simulink model "audio_dan"  (R2014a)
settings: Solver=FixedStepDiscrete  StartTime=0.0  StopTime=inf  FixedStep=0.00025  RelTol=1e-3
libraries: xpcethercatlib x12, slrtlib x4, simulink x1
settings Model: xpc_rtwmakecfg_data=_xpcethercatlib_  SimulationMode=external  BufferReuse=off  Creator=drl  LastModifiedBy=drl
settings SolverCC: EnableConcurrentExecution=on  ConcurrentTasks=on
settings OptimizationCC: BlockReduction=off  OptimizeBlockIOStorage=off  BufferReuse=off  GlobalBufferReuse=off  ExpressionFolding=off  LocalBlockOutputs=off
settings HardwareCC: ProdIntDivRoundTo=Zero  ProdEndianess=LittleEndian  ProdHWDeviceType=Generic->32-bit x86 compatible
settings RTWCC: SystemTargetFile=slrt.tlc  TemplateMakefile=slrt_default_tmf  Description=Simulink Real-Time  ProcessScript=slrt_make_rtw_hook  RTWCompilerOptimization=On
settings SimulinkRealTimeCC: GeneratePreprocessorConditionals=Disable all  EnableShiftOperators=on

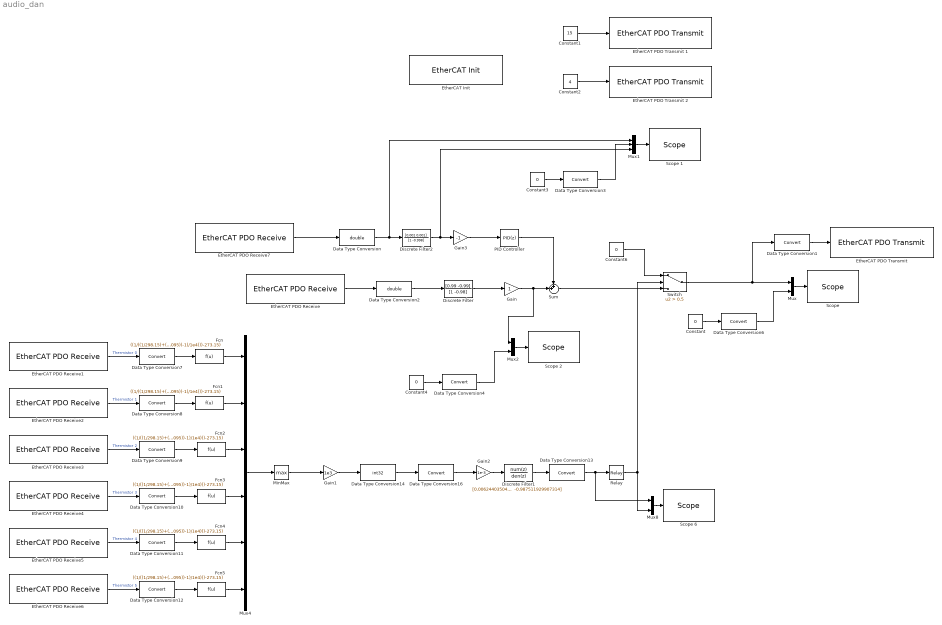
== system audio_dan ==
  Constant : Constant  Value=0  OutDataTypeStr=Inherit: Inherit via back propagation
  Constant1 : Constant  Value=15  OutDataTypeStr=Inherit: Inherit via back propagation  SampleTime=-1
  Constant2 : Constant  Value=4  OutDataTypeStr=Inherit: Inherit via back propagation  SampleTime=-1
  Constant3 : Constant  Value=0  OutDataTypeStr=Inherit: Inherit via back propagation
  Constant4 : Constant  Value=0  OutDataTypeStr=Inherit: Inherit via back propagation
  Constant6 : Constant  Value=0
  Data Type Conversion : DataTypeConversion  OutDataTypeStr=double
  Data Type Conversion{1,3..4,6..13,16} (12 alike) : DataTypeConversion
  Data Type Conversion14 : DataTypeConversion  OutDataTypeStr=int32
  Data Type Conversion2 : DataTypeConversion  OutDataTypeStr=double
  Discrete Filter : DiscreteFilter  Numerator=[0.99 -0.99]  Denominator=[1 -0.98]  a0EqualsOne=on
  Discrete Filter1 : DiscreteFilter  Numerator="[0.006244035046343   0.006244035046343]"  Denominator="[1.000000000000000  -0.987511929907314]"  a0EqualsOne=on
  Discrete Filter2 : DiscreteFilter  Numerator=[0.001 0.001]  Denominator=[1 -0.998]  a0EqualsOne=on
  "EtherCAT Init " : xpcethercatlib/EtherCAT Init   Priority=0  config_file=C:\Users\drl\Documents\MATLAB\eni_elmo_medulla_4khz.xml  device_id=0  pci_bus=4  pci_slot=0  enaDebug=on  enaDC=on  errLink=off  masterDbg=off  stateChgDbg=off  baseClock=off  masterCfg=off  logFile='c:\dbglog.txt'  sample_time=0.000250
  EtherCAT PDO Receive : xpcethercatlib/EtherCAT PDO Receive  Priority=2  sig_name=Drive 1 (Elmo Drive).Inputs.Analog Input 1  sig_offset=1144  sig_type=int16  type_size=16  sig_dim=1  device_id=0  sample_time=0.000250
  EtherCAT PDO Receive1 : xpcethercatlib/EtherCAT PDO Receive  Priority=2  sig_name=Box 2 (ATRIAS 2.1 Leg (Medulla 1.5)).Thermistors.Thermistor 0  sig_offset=808  sig_type=uint16  type_size=16  sig_dim=1  device_id=0  sample_time=0.000250
  EtherCAT PDO Receive2 : xpcethercatlib/EtherCAT PDO Receive  Priority=2  sig_name=Box 2 (ATRIAS 2.1 Leg (Medulla 1.5)).Thermistors.Thermistor 1  sig_offset=824  sig_type=uint16  type_size=16  sig_dim=1  device_id=0  sample_time=0.000250
  EtherCAT PDO Receive3 : xpcethercatlib/EtherCAT PDO Receive  Priority=2  sig_name=Box 2 (ATRIAS 2.1 Leg (Medulla 1.5)).Thermistors.Thermistor 2  sig_offset=840  sig_type=uint16  type_size=16  sig_dim=1  device_id=0  sample_time=0.000250
  EtherCAT PDO Receive4 : xpcethercatlib/EtherCAT PDO Receive  Priority=2  sig_name=Box 2 (ATRIAS 2.1 Leg (Medulla 1.5)).Thermistors.Thermistor 3  sig_offset=856  sig_type=uint16  type_size=16  sig_dim=1  device_id=0  sample_time=0.000250
  EtherCAT PDO Receive5 : xpcethercatlib/EtherCAT PDO Receive  Priority=2  sig_name=Box 2 (ATRIAS 2.1 Leg (Medulla 1.5)).Thermistors.Thermistor 4  sig_offset=872  sig_type=uint16  type_size=16  sig_dim=1  device_id=0  sample_time=0.000250
  EtherCAT PDO Receive6 : xpcethercatlib/EtherCAT PDO Receive  Priority=2  sig_name=Box 2 (ATRIAS 2.1 Leg (Medulla 1.5)).Thermistors.Thermistor 5  sig_offset=888  sig_type=uint16  type_size=16  sig_dim=1  device_id=0  sample_time=0.000250
  EtherCAT PDO Receive7 : xpcethercatlib/EtherCAT PDO Receive  Priority=2  sig_name=Drive 1 (Elmo Drive).Inputs.Position actual value  sig_offset=1064  sig_type=int32  type_size=32  sig_dim=1  device_id=0  sample_time=0.000250
  "EtherCAT PDO Transmit " : xpcethercatlib/EtherCAT PDO Transmit   Priority=3  sig_name=Drive 1 (Elmo Drive).Outputs.Target Torque  sig_offset=1064  sig_type=int16  type_size=16  sig_dim=1  device_id=0  sample_time=0.000250
  EtherCAT PDO Transmit 1 : xpcethercatlib/EtherCAT PDO Transmit   Priority=3  sig_name=Drive 1 (Elmo Drive).Outputs.Control word  sig_offset=1080  sig_type=uint16  type_size=16  sig_dim=1  device_id=0  sample_time=0.000250
  EtherCAT PDO Transmit 2 : xpcethercatlib/EtherCAT PDO Transmit   Priority=3  sig_name=Drive 1 (Elmo Drive).Outputs.Mode of operation  sig_offset=1096  sig_type=int8  type_size=8  sig_dim=1  device_id=0  sample_time=0.000250
  Fcn{,1..5} (6 alike) : Fcn  Expr=((1/((1/298.15)+(1/3988)*log(4700/((3.26/((u-172)*2.7/4095))-1)/1e4)))-273.15)
  Gain : Gain
  Gain1 : Gain  Gain=1e3
  Gain2 : Gain  Gain=1e-3
  Gain3 : Gain  Gain=-1
  MinMax : MinMax  Function=max
  Mux : Mux  Inputs=2
  Mux1 : Mux  Inputs=3
  Mux2 : Mux  Inputs=2
  Mux4 : Mux  Inputs=6
  Mux8 : Mux  Inputs=2
  PID Controller : simulink/Continuous/PID Controller  Controller=PID  TimeDomain=Discrete-time  SampleTime=-1  IntegratorMethod=Forward Euler  FilterMethod=Forward Euler  Form=Parallel  P=0.01  I=0  D=0.01  N=100  InitialConditionSource=internal  InitialConditionForIntegrator=0  InitialConditionForFilter=0  ExternalReset=none  LimitOutput=on  UpperSaturationLimit=200  LowerSaturationLimit=-200  LinearizeAsGain=on  AntiWindupMode=none  Kb=1  TrackingMode=off  Kt=1  PParamMin=[]  PParamMax=[]  IParamMin=[]  IParamMax=[]  DParamMin=[]  DParamMax=[]  NParamMin=[]  NParamMax=[]  KbParamMin=[]  KbParamMax=[]  KtParamMin=[]  KtParamMax=[]  POutMin=[]  POutMax=[]  IOutMin=[]  IOutMax=[]  DOutMin=[]  DOutMax=[]  NOutMin=[]  NOutMax=[]  KbOutMin=[]  KbOutMax=[]  KtOutMin=[]  KtOutMax=[]  IntegratorOutMin=[]  IntegratorOutMax=[]  FilterOutMin=[]  FilterOutMax=[]  SumOutMin=[]  SumOutMax=[]  SumI1OutMin=[]  SumI1OutMax=[]  SumI2OutMin=[]  SumI2OutMax=[]  SumI3OutMin=[]  SumI3OutMax=[]  SumDOutMin=[]  SumDOutMax=[]  SaturationOutMin=[]  SaturationOutMax=[]  IntegratorContinuousStateAttributes=''  IntegratorStateMustResolveToSignalObject=off  IntegratorRTWStateStorageClass=Auto  FilterContinuousStateAttributes=''  FilterStateMustResolveToSignalObject=off  FilterRTWStateStorageClass=Auto
  Relay : Relay  OnSwitchValue=80  OffSwitchValue=60
  "Scope " : slrtlib/Displays and Logging/Scope   scopeno=1  scopetype=Target  autostart=on  viewmode=Graphical rolling  formatstr='%15.6f'  grid=on  ylimits=[0,0]  nosamples=1000  noprepostsamples=0  interleave=1  triggermode=FreeRun  triggersignal=1  trigsignalfromport=off  triggerlevel=0.0  triggerslope=Either  triggerscope=1  triggersample=0  filename=data.dat  mode=Lazy  writesize=512  autorestart=off  dynamicfilemode=off  maxwritefilesize=512*1024^2
  Scope 1 : slrtlib/Displays and Logging/Scope   scopeno=3  scopetype=Target  autostart=on  viewmode=Graphical rolling  formatstr='%15.6f'  grid=on  ylimits=[0,0]  nosamples=1000  noprepostsamples=0  interleave=1  triggermode=FreeRun  triggersignal=1  trigsignalfromport=off  triggerlevel=0.0  triggerslope=Either  triggerscope=1  triggersample=0  filename=data.dat  mode=Lazy  writesize=512  autorestart=off  dynamicfilemode=off  maxwritefilesize=512*1024^2
  Scope 2 : slrtlib/Displays and Logging/Scope   scopeno=4  scopetype=Target  autostart=on  viewmode=Graphical rolling  formatstr='%15.6f'  grid=on  ylimits=[0,0]  nosamples=1000  noprepostsamples=0  interleave=1  triggermode=FreeRun  triggersignal=1  trigsignalfromport=off  triggerlevel=0.0  triggerslope=Either  triggerscope=1  triggersample=0  filename=data.dat  mode=Lazy  writesize=512  autorestart=off  dynamicfilemode=off  maxwritefilesize=512*1024^2
  Scope 6 : slrtlib/Displays and Logging/Scope   scopeno=2  scopetype=Target  autostart=on  viewmode=Numerical  formatstr='%f'  grid=on  ylimits=[0,0]  nosamples=100  noprepostsamples=0  interleave=1  triggermode=FreeRun  triggersignal=1  trigsignalfromport=off  triggerlevel=0.0  triggerslope=Either  triggerscope=2  triggersample=0  filename=data.dat  mode=Lazy  writesize=512  autorestart=off  dynamicfilemode=off  maxwritefilesize=512*1024^2
  Sum : Sum  Inputs=++|
  Switch : Switch  Criteria=u2 > Threshold  Threshold=0.5
  wires:
  Mux/1 -> "Scope "/1
  Data Type Conversion1/1 -> "EtherCAT PDO Transmit "/1
  Constant1/1 -> EtherCAT PDO Transmit 1/1
  Constant2/1 -> EtherCAT PDO Transmit 2/1
  EtherCAT PDO Receive6/1 -> Data Type Conversion12/1  "Thermistor 5"
  EtherCAT PDO Receive5/1 -> Data Type Conversion11/1  "Thermistor 4"
  EtherCAT PDO Receive4/1 -> Data Type Conversion10/1  "Thermistor 3"
  EtherCAT PDO Receive3/1 -> Data Type Conversion9/1  "Thermistor 2"
  EtherCAT PDO Receive2/1 -> Data Type Conversion8/1  "Thermistor 1"
  EtherCAT PDO Receive1/1 -> Data Type Conversion7/1  "Thermistor 0"
  Data Type Conversion7/1 -> Fcn/1
  Fcn/1 -> Mux4/1
  Data Type Conversion12/1 -> Fcn5/1
  Data Type Conversion11/1 -> Fcn4/1
  Data Type Conversion10/1 -> Fcn3/1
  Data Type Conversion9/1 -> Fcn2/1
  Data Type Conversion8/1 -> Fcn1/1
  Fcn1/1 -> Mux4/2
  Fcn2/1 -> Mux4/3
  Fcn3/1 -> Mux4/4
  Fcn4/1 -> Mux4/5
  Fcn5/1 -> Mux4/6
  Data Type Conversion13/1 -> Mux8/1, Relay/1
  Mux8/1 -> Scope 6/1
  Discrete Filter1/1 -> Data Type Conversion13/1
  Gain2/1 -> Discrete Filter1/1
  MinMax/1 -> Gain1/1
  Gain1/1 -> Data Type Conversion14/1
  Data Type Conversion14/1 -> Data Type Conversion16/1
  Data Type Conversion16/1 -> Gain2/1
  Mux4/1 -> MinMax/1
  Constant6/1 -> Switch/1
  Relay/1 -> Switch/2, Mux8/2
  Gain/1 -> Mux2/1, Sum/2
  Sum/1 -> Switch/3
  Switch/1 -> Data Type Conversion1/1, Mux/1
  Constant/1 -> Data Type Conversion6/1
  Data Type Conversion6/1 -> Mux/2
  PID Controller/1 -> Sum/1
  Constant3/1 -> Data Type Conversion3/1
  Data Type Conversion3/1 -> Mux1/2
  Mux1/1 -> Scope 1/1
  Constant4/1 -> Data Type Conversion4/1
  Data Type Conversion4/1 -> Mux2/2
  Mux2/1 -> Scope 2/1
  EtherCAT PDO Receive7/1 -> Data Type Conversion/1
  Gain3/1 -> PID Controller/1
  Data Type Conversion/1 -> Mux1/1, Discrete Filter2/1
  Discrete Filter2/1 -> Mux1/3, Gain3/1
  EtherCAT PDO Receive/1 -> Data Type Conversion2/1
  Data Type Conversion2/1 -> Discrete Filter/1
  Discrete Filter/1 -> Gain/1
